simulink model "func_demo"  (R2020b)
settings: Solver=VariableStepAuto  StartTime=0.0  StopTime=10.0  RelTol=1e-3
settings Model: Creator=Training  LastModifiedBy=Training

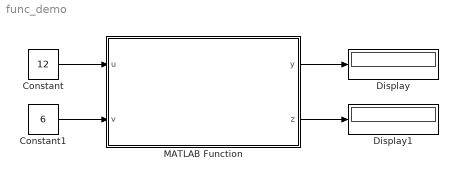
== system func_demo ==
  Constant : Constant  Value=12
  Constant1 : Constant  Value=6
  Display : Display
  Display1 : Display
  MATLAB Function : MATLAB Function  TreatAsAtomicUnit=on
  wires:
  Constant/1 -> MATLAB Function/1(u)
  MATLAB Function/1(y) -> Display/1
  Constant1/1 -> MATLAB Function/2(v)
  MATLAB Function/2(z) -> Display1/1

== matlab function func_demo/MATLAB Function ==
  data: u input; y output; v input; z output
function [y,z] = fcn(u,v)

y = u*v;
z = u+v;
